simulink model "Continuos_Vs_Discrete"  (R2025a)
settings: Solver=VariableStepAuto  StartTime=0.0  StopTime=0.7  RelTol=1e-3
settings Model: Creator=Eduardoht  LastModifiedBy=Eduardoht

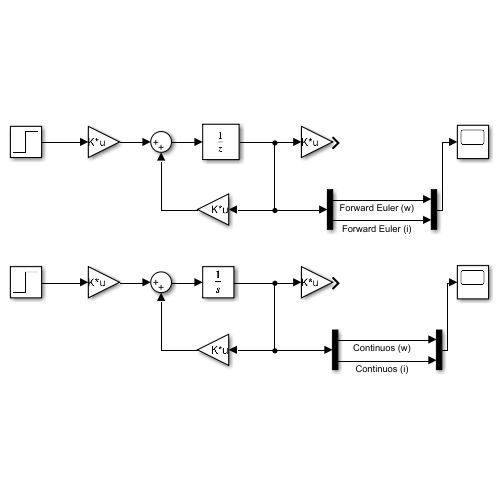
[thumbnail: Simulink's stored preview of the top-level diagram]
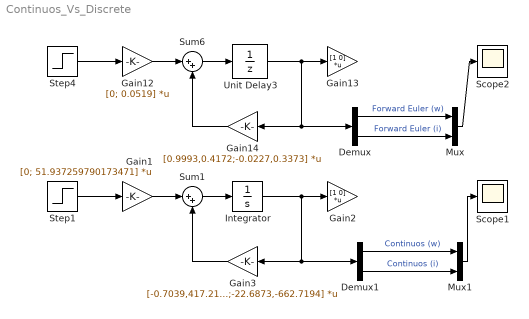
== system Continuos_Vs_Discrete ==
  Demux : Demux  Outputs=2
  Demux1 : Demux  Outputs=2
  Gain1 : Gain  Gain=[0; 51.937259790173471]  Multiplication=Matrix(K*u)
  Gain12 : Gain  Gain=[0; 0.0519]  Multiplication=Matrix(K*u)
  Gain13 : Gain  Gain=[1 0]  Multiplication=Matrix(K*u)
  Gain14 : Gain  Gain=[0.9993,0.4172;-0.0227,0.3373]  Multiplication=Matrix(K*u)
  Gain2 : Gain  Gain=[1 0]  Multiplication=Matrix(K*u)
  Gain3 : Gain  Gain=[-0.7039,417.2130;-22.6873,-662.7194]  Multiplication=Matrix(K*u)
  Integrator : Integrator
  Mux : Mux  Inputs=2
  Mux1 : Mux  Inputs=2
  Scope1 : Scope
      settings: ActiveDisplayYMinimum=-0.27244766380821739  ActiveDisplayYMaximum=2.4520289742739569
  Scope2 : Scope
      settings: ActiveDisplayYMinimum=-0.27244766380821739  ActiveDisplayYMaximum=2.4520289742739569
  Step1 : Step  Time=0  SampleTime=0
  Step4 : Step  Time=0  SampleTime=0
  Sum1 : Sum  Inputs=|++
  Sum6 : Sum  Inputs=|++
  Unit Delay3 : UnitDelay  InitialCondition=[0; 0];  SampleTime=0.001  HasFrameUpgradeWarning=on
  wires:
  Step4/1 -> Gain12/1
  Gain12/1 -> Sum6/1
  Gain14/1 -> Sum6/2
  Sum6/1 -> Unit Delay3/1
  Step1/1 -> Gain1/1
  Sum1/1 -> Integrator/1
  Gain1/1 -> Sum1/1
  Gain3/1 -> Sum1/2
  Unit Delay3/1 -> Demux/1, Gain14/1, Gain13/1
  Demux/1 -> Mux/1  "Forward Euler (w)"
  Demux/2 -> Mux/2  "Forward Euler (i)"
  Mux/1 -> Scope2/1
  Demux1/1 -> Mux1/1  "Continuos (w)"
  Mux1/1 -> Scope1/1
  Integrator/1 -> Demux1/1, Gain3/1, Gain2/1
  Demux1/2 -> Mux1/2  "Continuos (i)"
